simulink model "noPattern"  (R2020a)
settings: Solver=VariableStepAuto  StartTime=0.0  StopTime=0.5  RelTol=1e-3
model workspace (MAT data in the model file):
  Ts = 0.1
libraries: simulink x1
settings Model: Creator=liuzhenjie  LastModifiedBy=liuzhenjie

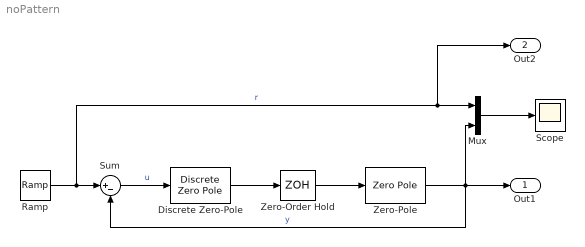
== system noPattern ==
  Discrete Zero-Pole : DiscreteZeroPole  Zeros=|  Poles=|  Gain=52.3666  SampleTime=Ts
      Zeros=|
      | [
      |     0.9048
      |     0.5987]
      Poles=|
      | [   -0.7334
      |     1.0000]
  Mux : Mux  Inputs=2
  Ramp : simulink/Sources/Ramp  slope=1  start=0  InitialOutput=0
  Scope : Scope
  Sum : Sum  Inputs=|+-
  Zero-Order Hold : ZeroOrderHold  SampleTime=Ts
  Zero-Pole : ZeroPole  Zeros=[]  Poles=[0 -1]  Gain=5
  Out1 : Outport
  Out2 : Outport  Port=2
  wires:
  Mux/1 -> Scope/1
  Sum/1 -> Discrete Zero-Pole/1  "u"
  Zero-Pole/1 -> Mux/2, Sum/2, Out1/1  "y"
  Discrete Zero-Pole/1 -> Zero-Order Hold/1
  Zero-Order Hold/1 -> Zero-Pole/1
  Ramp/1 -> Out2/1, Mux/1, Sum/1  "r"
